simulink model "AB_Final_of_MPC_Bandwidth_Result_UnbalancedNew"  (R2022b)
settings: Solver=FixedStepDiscrete  StartTime=0.0  StopTime=Inf  FixedStep=100e-6  RelTol=1e-3  EnableMultiTasking=on
undefined symbols (not defined in the file): C28x, CPU1, CPU2, CurrentBypassValue, DiscIntNeverNeededParam, Down, GPTRIP1SEL, TZ1, Up
libraries: c2802xlib x20, simulink x17, dspstat3 x13, eeGeneralControl x10, c2837xDlib x5, c280xlib x5, PID_Lib x4, c2000lib x1, spsAlphaBetaZerotoabcLib x1
(part 4 of 10)

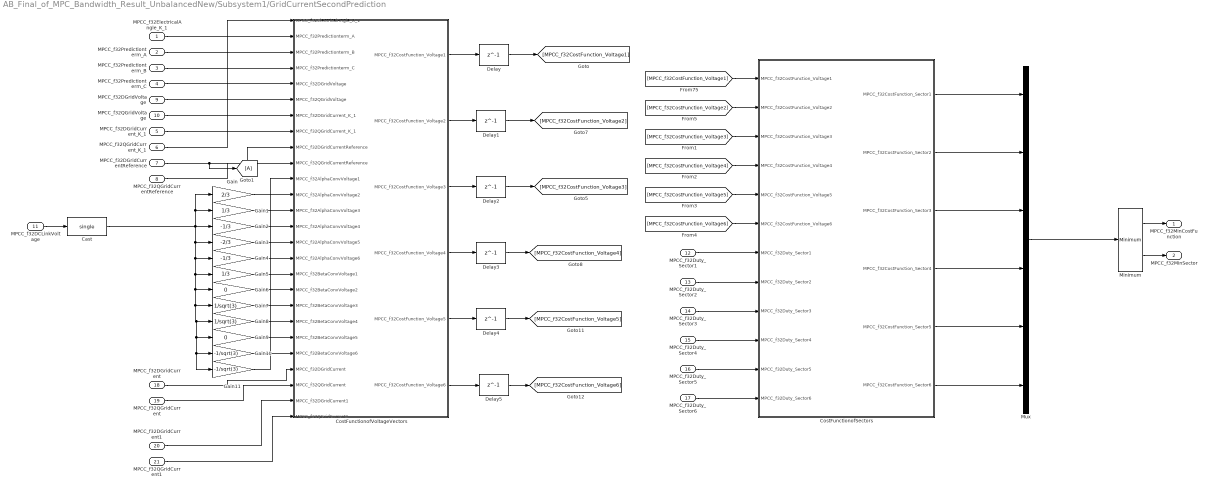
== system AB_Final_of_MPC_Bandwidth_Result_UnbalancedNew/Subsystem1/GridCurrentSecondPrediction ==
  MPCC_f32ElectricalAngle_K_1 : Inport
  MPCC_f32Predictionterm_A : Inport  Port=2
  MPCC_f32Predictionterm_B : Inport  Port=3
  MPCC_f32Predictionterm_C : Inport  Port=4
  MPCC_f32DGridCurrent_K_1 : Inport  Port=5
  MPCC_f32QGridCurrent_K_1 : Inport  Port=6
  MPCC_f32DGridCurrentReference : Inport  Port=7
  MPCC_f32QGridCurrentReference : Inport  Port=8
  MPCC_f32DGridVoltage : Inport  Port=9
  MPCC_f32QGridVoltage : Inport  Port=10
  MPCC_f32DCLinkVoltage : Inport  Port=11
  MPCC_f32Duty_Sector1 : Inport  Port=12
  MPCC_f32Duty_Sector2 : Inport  Port=13
  MPCC_f32Duty_Sector3 : Inport  Port=14
  MPCC_f32Duty_Sector4 : Inport  Port=15
  MPCC_f32Duty_Sector5 : Inport  Port=16
  MPCC_f32Duty_Sector6 : Inport  Port=17
  MPCC_f32DGridCurrent : Inport  Port=18
  MPCC_f32QGridCurrent : Inport  Port=19
  MPCC_f32DGridCurrent1 : Inport  Port=20
  MPCC_f32QGridCurrent1 : Inport  Port=21
  Cast : DataTypeConversion  OutDataTypeStr=single  SaturateOnIntegerOverflow=off  RndMeth=Floor
  CostFunctionofSectors : Subsystem
  CostFunctionofVoltageVectors : Subsystem
  Delay{,1..5} (6 alike) : Delay  DelayLength=1  InitialCondition=single(1000000)  UseCircularBuffer=on
  Gain : Gain  Gain=2/3
  Gain1 : Gain  Gain=1/3
  Gain10 : Gain  Gain=-1/sqrt(3)
  Gain11 : Gain  Gain=-1/sqrt(3)
  Gain2 : Gain  Gain=-1/3
  Gain3 : Gain  Gain=-2/3
  Gain4 : Gain  Gain=-1/3
  Gain5 : Gain  Gain=1/3
  Gain6 : Gain  Gain=0
  Gain7 : Gain  Gain=1/sqrt(3)
  Gain8 : Gain  Gain=1/sqrt(3)
  Gain9 : Gain  Gain=0
  Goto1 : Goto
  Minimum : dspstat3/Minimum  operation=minimum  fcn=Value and Index  indexBase=One  operateOver=Each column  Dimension=1  InputProcessing=Columns as channels (frame based)  reset=None  roiEnable=off  roiType=Rectangles  roiPortion=Entire ROI  roiOutput=Individual statistics for each ROI  roiFlag=off  roundingMode=Floor  overflowMode=off
  Mux : Mux  Inputs=6
  MPCC_f32MinCostFunction : Outport
  MPCC_f32MinSector : Outport  Port=2
  wires:
  CostFunctionofVoltageVectors/3(MPCC_f32CostFunction_Voltage3) -> Delay2/1
  CostFunctionofVoltageVectors/2(MPCC_f32CostFunction_Voltage2) -> Delay1/1
  CostFunctionofVoltageVectors/5(MPCC_f32CostFunction_Voltage5) -> Delay4/1
  CostFunctionofVoltageVectors/6(MPCC_f32CostFunction_Voltage6) -> Delay5/1
  CostFunctionofVoltageVectors/4(MPCC_f32CostFunction_Voltage4) -> Delay3/1
  CostFunctionofVoltageVectors/1(MPCC_f32CostFunction_Voltage1) -> Delay/1
  MPCC_f32ElectricalAngle_K_1/1 -> CostFunctionofVoltageVectors/1(MPCC_f32ElectricalAngle_K_1)
  MPCC_f32Predictionterm_A/1 -> CostFunctionofVoltageVectors/2(MPCC_f32Predictionterm_A)
  MPCC_f32Predictionterm_B/1 -> CostFunctionofVoltageVectors/3(MPCC_f32Predictionterm_B)
  MPCC_f32Predictionterm_C/1 -> CostFunctionofVoltageVectors/4(MPCC_f32Predictionterm_C)
  MPCC_f32DGridVoltage/1 -> CostFunctionofVoltageVectors/5(MPCC_f32DGridVoltage)
  MPCC_f32QGridVoltage/1 -> CostFunctionofVoltageVectors/6(MPCC_f32QGridVoltage)
  MPCC_f32DGridCurrent_K_1/1 -> CostFunctionofVoltageVectors/7(MPCC_f32DGridCurrent_K_1)
  MPCC_f32QGridCurrent_K_1/1 -> CostFunctionofVoltageVectors/8(MPCC_f32QGridCurrent_K_1)
  MPCC_f32DGridCurrentReference/1 -> Goto1/1, CostFunctionofVoltageVectors/9(MPCC_f32DGridCurrentReference)
  MPCC_f32QGridCurrentReference/1 -> CostFunctionofVoltageVectors/10(MPCC_f32QGridCurrentReference)
  MPCC_f32DCLinkVoltage/1 -> Cast/1
  Gain/1 -> CostFunctionofVoltageVectors/11(MPCC_f32AlphaConvVoltage1)
  Gain1/1 -> CostFunctionofVoltageVectors/12(MPCC_f32AlphaConvVoltage2)
  Gain2/1 -> CostFunctionofVoltageVectors/13(MPCC_f32AlphaConvVoltage3)
  Gain3/1 -> CostFunctionofVoltageVectors/14(MPCC_f32AlphaConvVoltage4)
  Gain4/1 -> CostFunctionofVoltageVectors/15(MPCC_f32AlphaConvVoltage5)
  Gain5/1 -> CostFunctionofVoltageVectors/16(MPCC_f32AlphaConvVoltage6)
  Gain6/1 -> CostFunctionofVoltageVectors/17(MPCC_f32BetaConvVoltage1)
  Gain7/1 -> CostFunctionofVoltageVectors/18(MPCC_f32BetaConvVoltage2)
  Gain8/1 -> CostFunctionofVoltageVectors/19(MPCC_f32BetaConvVoltage3)
  Gain9/1 -> CostFunctionofVoltageVectors/20(MPCC_f32BetaConvVoltage4)
  Gain10/1 -> CostFunctionofVoltageVectors/21(MPCC_f32BetaConvVoltage5)
  Gain11/1 -> CostFunctionofVoltageVectors/22(MPCC_f32BetaConvVoltage6)
  [MPCC_f32CostFunction_Voltage1] -> CostFunctionofSectors/1(MPCC_f32CostFunction_Voltage1)
  [MPCC_f32CostFunction_Voltage4] -> CostFunctionofSectors/4(MPCC_f32CostFunction_Voltage4)
  [MPCC_f32CostFunction_Voltage5] -> CostFunctionofSectors/5(MPCC_f32CostFunction_Voltage5)
  [MPCC_f32CostFunction_Voltage6] -> CostFunctionofSectors/6(MPCC_f32CostFunction_Voltage6)
  [MPCC_f32CostFunction_Voltage2] -> CostFunctionofSectors/2(MPCC_f32CostFunction_Voltage2)
  [MPCC_f32CostFunction_Voltage3] -> CostFunctionofSectors/3(MPCC_f32CostFunction_Voltage3)
  CostFunctionofSectors/1(MPCC_f32CostFunction_Sector1) -> Mux/1
  CostFunctionofSectors/2(MPCC_f32CostFunction_Sector2) -> Mux/2
  CostFunctionofSectors/3(MPCC_f32CostFunction_Sector3) -> Mux/3
  CostFunctionofSectors/4(MPCC_f32CostFunction_Sector4) -> Mux/4
  CostFunctionofSectors/5(MPCC_f32CostFunction_Sector5) -> Mux/5
  CostFunctionofSectors/6(MPCC_f32CostFunction_Sector6) -> Mux/6
  Mux/1 -> Minimum/1
  MPCC_f32Duty_Sector1/1 -> CostFunctionofSectors/7(MPCC_f32Duty_Sector1)
  MPCC_f32Duty_Sector2/1 -> CostFunctionofSectors/8(MPCC_f32Duty_Sector2)
  MPCC_f32Duty_Sector3/1 -> CostFunctionofSectors/9(MPCC_f32Duty_Sector3)
  MPCC_f32Duty_Sector4/1 -> CostFunctionofSectors/10(MPCC_f32Duty_Sector4)
  MPCC_f32Duty_Sector5/1 -> CostFunctionofSectors/11(MPCC_f32Duty_Sector5)
  MPCC_f32Duty_Sector6/1 -> CostFunctionofSectors/12(MPCC_f32Duty_Sector6)
  Cast/1 -> Gain4/1, Gain9/1, Gain11/1, Gain10/1, Gain8/1, Gain7/1, Gain6/1, Gain5/1, Gain3/1, Gain/1, Gain1/1, Gain2/1
  Delay/1 -> [MPCC_f32CostFunction_Voltage1]
  Delay1/1 -> [MPCC_f32CostFunction_Voltage2]
  Delay2/1 -> [MPCC_f32CostFunction_Voltage3]
  Delay3/1 -> [MPCC_f32CostFunction_Voltage4]
  Delay4/1 -> [MPCC_f32CostFunction_Voltage5]
  Delay5/1 -> [MPCC_f32CostFunction_Voltage6]
  MPCC_f32QGridCurrent/1 -> CostFunctionofVoltageVectors/24(MPCC_f32QGridCurrent)
  MPCC_f32DGridCurrent/1 -> CostFunctionofVoltageVectors/23(MPCC_f32DGridCurrent)
  Minimum/1 -> MPCC_f32MinCostFunction/1
  Minimum/2 -> MPCC_f32MinSector/1
  MPCC_f32DGridCurrent1/1 -> CostFunctionofVoltageVectors/25(MPCC_f32DGridCurrent1)
  MPCC_f32QGridCurrent1/1 -> CostFunctionofVoltageVectors/26(MPCC_f32QGridCurrent1)

== system AB_Final_of_MPC_Bandwidth_Result_UnbalancedNew/Subsystem1/ModulatorTimes ==
  MPCC_f32ElectricalAngle_K_1 : Inport
  MPCC_f32DCLinkVoltage : Inport  Port=2
  MPCC_f32Duty_Sector1 : Inport  Port=3
  MPCC_f32Duty_Sector2 : Inport  Port=4
  MPCC_f32Duty_Sector3 : Inport  Port=5
  MPCC_f32Duty_Sector4 : Inport  Port=6
  MPCC_f32Duty_Sector5 : Inport  Port=7
  MPCC_f32Duty_Sector6 : Inport  Port=8
  MPCC_f32MinSector : Inport  Port=9
  MPCC_f32SwitchingPeriod : Inport  Port=10
  Cast : DataTypeConversion  OutDataTypeStr=single  SaturateOnIntegerOverflow=off  RndMeth=Floor
  ConverterVoltage : Subsystem
  Gain : Gain  Gain=2/3
  Gain1 : Gain  Gain=1/3
  Gain10 : Gain  Gain=-1/sqrt(3)
  Gain11 : Gain  Gain=-1/sqrt(3)
  Gain2 : Gain  Gain=-1/3
  Gain3 : Gain  Gain=-2/3
  Gain4 : Gain  Gain=-1/3
  Gain5 : Gain  Gain=1/3
  Gain6 : Gain  Gain=0
  Gain7 : Gain  Gain=1/sqrt(3)
  Gain8 : Gain  Gain=1/sqrt(3)
  Gain9 : Gain  Gain=0
  ModulationVectorTimes : Subsystem
  MPCC_f32DQConvVoltage : Outport
  MPCC_f32Time1 : Outport  Port=2
  MPCC_f32Time2 : Outport  Port=3
  MPCC_f32Time0 : Outport  Port=4
  MPCC_u8ModulationSector : Outport  Port=5
  wires:
  MPCC_f32ElectricalAngle_K_1/1 -> ConverterVoltage/1(MPCC_f32ElectricalAngle_K_1)
  MPCC_f32DCLinkVoltage/1 -> Cast/1
  Gain/1 -> ConverterVoltage/2(MPCC_f32AlphaConvVoltage1)
  Gain1/1 -> ConverterVoltage/3(MPCC_f32AlphaConvVoltage2)
  Gain2/1 -> ConverterVoltage/4(MPCC_f32AlphaConvVoltage3)
  Gain3/1 -> ConverterVoltage/5(MPCC_f32AlphaConvVoltage4)
  Gain4/1 -> ConverterVoltage/6(MPCC_f32AlphaConvVoltage5)
  Gain5/1 -> ConverterVoltage/7(MPCC_f32AlphaConvVoltage6)
  Gain6/1 -> ConverterVoltage/8(MPCC_f32BetaConvVoltage1)
  Gain7/1 -> ConverterVoltage/9(MPCC_f32BetaConvVoltage2)
  Gain8/1 -> ConverterVoltage/10(MPCC_f32BetaConvVoltage3)
  Gain9/1 -> ConverterVoltage/11(MPCC_f32BetaConvVoltage4)
  Gain10/1 -> ConverterVoltage/12(MPCC_f32BetaConvVoltage5)
  Gain11/1 -> ConverterVoltage/13(MPCC_f32BetaConvVoltage6)
  ConverterVoltage/1(MPCC_f32DQConvVoltage) -> MPCC_f32DQConvVoltage/1
  MPCC_f32Duty_Sector5/1 -> [MPCC_f32Duty_Sector5]
  MPCC_f32Duty_Sector1/1 -> [MPCC_f32Duty_Sector1]
  MPCC_f32Duty_Sector6/1 -> [MPCC_f32Duty_Sector6]
  MPCC_f32Duty_Sector2/1 -> [MPCC_f32Duty_Sector2]
  MPCC_f32Duty_Sector4/1 -> [MPCC_f32Duty_Sector4]
  MPCC_f32Duty_Sector3/1 -> [MPCC_f32Duty_Sector3]
  MPCC_f32MinSector/1 -> [MPCC_f32MinSector], ConverterVoltage/20(MPCC_f32MinSector)
  [MPCC_f32Duty_Sector6] -> ConverterVoltage/19(MPCC_f32Duty_Sector6)
  [MPCC_f32Duty_Sector5] -> ConverterVoltage/18(MPCC_f32Duty_Sector5)
  [MPCC_f32Duty_Sector1] -> ConverterVoltage/14(MPCC_f32Duty_Sector1)
  [MPCC_f32Duty_Sector2] -> ConverterVoltage/15(MPCC_f32Duty_Sector2)
  [MPCC_f32Duty_Sector3] -> ConverterVoltage/16(MPCC_f32Duty_Sector3)
  [MPCC_f32Duty_Sector4] -> ConverterVoltage/17(MPCC_f32Duty_Sector4)
  [MPCC_f32Duty_Sector1] -> ModulationVectorTimes/1(MPCC_f32Duty_Sector1)
  [MPCC_f32Duty_Sector2] -> ModulationVectorTimes/2(MPCC_f32Duty_Sector2)
  [MPCC_f32Duty_Sector3] -> ModulationVectorTimes/3(MPCC_f32Duty_Sector3)
  [MPCC_f32Duty_Sector4] -> ModulationVectorTimes/4(MPCC_f32Duty_Sector4)
  [MPCC_f32Duty_Sector5] -> ModulationVectorTimes/5(MPCC_f32Duty_Sector5)
  [MPCC_f32Duty_Sector6] -> ModulationVectorTimes/6(MPCC_f32Duty_Sector6)
  MPCC_f32SwitchingPeriod/1 -> ModulationVectorTimes/7(MPCC_f32SwitchingPeriod)
  [MPCC_f32MinSector] -> ModulationVectorTimes/8(MPCC_f32MinSector)
  ModulationVectorTimes/3(MPCC_f32Time0) -> MPCC_f32Time0/1
  ModulationVectorTimes/1(MPCC_f32Time1) -> MPCC_f32Time1/1
  ModulationVectorTimes/2(MPCC_f32Time2) -> MPCC_f32Time2/1
  ModulationVectorTimes/4(MPCC_u8ModulationSector) -> MPCC_u8ModulationSector/1
  Cast/1 -> Gain/1, Gain4/1, Gain9/1, Gain11/1, Gain10/1, Gain8/1, Gain7/1, Gain6/1, Gain5/1, Gain3/1, Gain2/1, Gain1/1

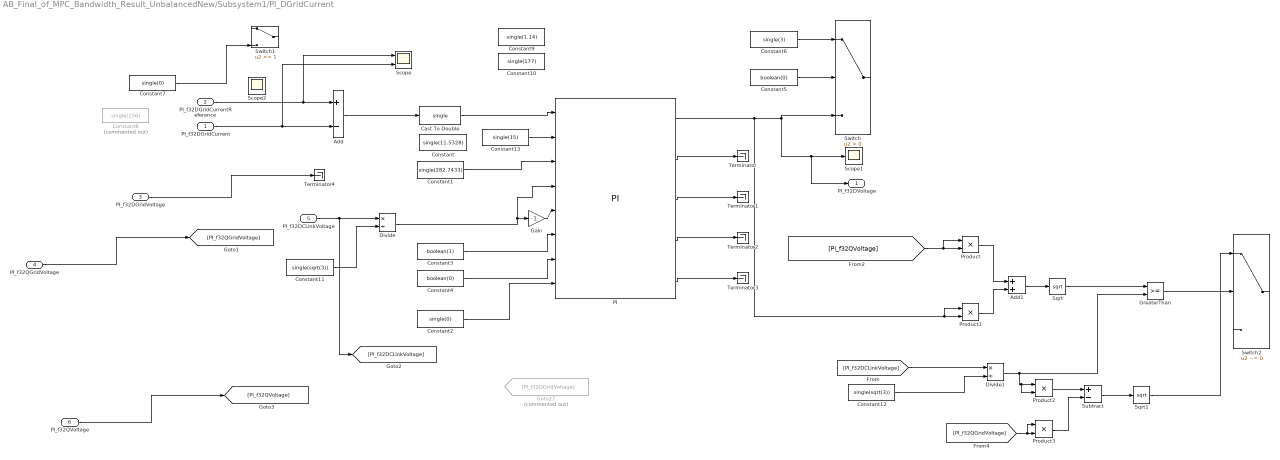
== system AB_Final_of_MPC_Bandwidth_Result_UnbalancedNew/Subsystem1/PI_DGridCurrent ==
  PI_f32DGridCurrent : Inport
  PI_f32DGridCurrentReference : Inport  Port=2
  PI_f32DGridVoltage : Inport  Port=3
  PI_f32QGridVoltage : Inport  Port=4
  PI_f32DCLinkVoltage : Inport  Port=5
  PI_f32QVoltage : Inport  Port=6
  Add : Sum  Inputs=+-
  Add1 : Sum
  Cast To Double : DataTypeConversion  OutDataTypeStr=single  SaturateOnIntegerOverflow=off  RndMeth=Floor
  Constant : Constant  Value=single(11.5328)
  Constant1 : Constant  Value=single(282.7433)
  Constant10 : Constant  Value=single(177)
  Constant11 : Constant  Value=single(sqrt(3))
  Constant12 : Constant  Value=single(sqrt(3))
  Constant13 : Constant  Value=single(15)
  Constant2 : Constant  Value=single(0)
  Constant3 : Constant  Value=boolean(1)
  Constant4 : Constant  Value=boolean(0)
  Constant5 : Constant  Value=boolean(0)
  Constant6 : Constant  Value=single(3)
  Constant7 : Constant  Value=single(0)
  Constant8 : Constant  Commented=on  Value=single(156)
  Constant9 : Constant  Value=single(1.14)
  Divide : Product  Inputs=*/  RndMeth=Zero  SaturateOnIntegerOverflow=on
  Divide1 : Product  Inputs=*/  RndMeth=Zero  SaturateOnIntegerOverflow=on
  Gain : Gain  Gain=-1
  Goto27 : Goto  Commented=on  GotoTag=PI_f32DGridVoltage
  GreaterThan : RelationalOperator  OutDataTypeStr=boolean  RndMeth=Simplest  InputSameDT=off
  PI : PID_Lib/PI  SystemSampleTime=-1  VariantActivationTime=update diagram  Latency=0  AutoFrameSizeCalculation=off
  Product{,1..3} (4 alike) : Product
  Scope : Scope  NumInputPorts=2
  Scope1 : Scope
  Scope2 : Scope
  Sqrt : Sqrt
  Sqrt1 : Sqrt
  Subtract : Sum  Inputs=+-
  Switch : Switch  Criteria=u2 > Threshold  SaturateOnIntegerOverflow=off  InputSameDT=off
  Switch1 : Switch  Threshold=1  SaturateOnIntegerOverflow=off  InputSameDT=off
  Switch2 : Switch  Criteria=u2 ~= 0  SaturateOnIntegerOverflow=off  InputSameDT=off
  Terminator{,1..4} (5 alike) : Terminator
  PI_f32DVoltage : Outport
  wires:
  PI_f32DGridCurrent/1 -> Scope/2, Add/2
  Gain/1 -> PI/5
  Constant3/1 -> PI/6
  Constant4/1 -> PI/7
  PI/2 -> Terminator/1
  PI/3 -> Terminator1/1
  PI/4 -> Terminator2/1
  PI/5 -> Terminator3/1
  Constant5/1 -> Switch/2
  Constant6/1 -> Switch/1
  Cast To Double/1 -> PI/1
  Add/1 -> Cast To Double/1
  Constant7/1 -> Switch1/3
  PI_f32DGridCurrentReference/1 -> Scope/1, Add/1
  Constant2/1 -> PI/8
  PI_f32DGridVoltage/1 -> Terminator4/1
  PI_f32QGridVoltage/1 -> [PI_f32QGridVoltage]
  Add1/1 -> Sqrt/1
  Product1/1 -> Add1/2
  Product/1 -> Add1/1
  [PI_f32QVoltage] -> Product/1, Product/2
  PI/1 -> Product1/1, Product1/2, Switch/3, PI_f32DVoltage/1, Scope1/1
  PI_f32DCLinkVoltage/1 -> [PI_f32DCLinkVoltage], Divide/1
  Constant11/1 -> Divide/2
  Constant12/1 -> Divide1/2
  [PI_f32DCLinkVoltage] -> Divide1/1
  Sqrt/1 -> GreaterThan/1
  Divide1/1 -> Product2/2, Product2/1, GreaterThan/2
  GreaterThan/1 -> Switch2/2
  Product2/1 -> Subtract/1
  [PI_f32QGridVoltage] -> Product3/1, Product3/2
  Product3/1 -> Subtract/2
  Subtract/1 -> Sqrt1/1
  Sqrt1/1 -> Switch2/1
  Divide/1 -> PI/4, Gain/1
  PI_f32QVoltage/1 -> [PI_f32QVoltage]
  Constant1/1 -> PI/3
  Constant13/1 -> PI/2

== system AB_Final_of_MPC_Bandwidth_Result_UnbalancedNew/Subsystem1/PI_QGridCurrent ==
  PI_f32QGridCurrentReference : Inport
  PI_f32QGridCurrent : Inport  Port=2
  PI_f32QGridVoltage : Inport  Port=3
  PI_f32DGridVoltage : Inport  Port=4
  PI_f32DCLinkVoltage : Inport  Port=5
  Add : Sum  Inputs=+-
  Add1 : Sum
  Cast To Single : DataTypeConversion  OutDataTypeStr=single  SaturateOnIntegerOverflow=off  RndMeth=Floor
  Constant : Constant  Value=single(11.5328)
  Constant1 : Constant  Value=single(282.7433)
  Constant10 : Constant  Value=single(177)
  Constant11 : Constant  Value=single(sqrt(3))
  Constant12 : Constant  Value=single(1.14)
  Constant13 : Constant  Value=single(sqrt(3))
  Constant14 : Constant  Value=single(15)
  Constant2 : Constant  Value=single(156)
  Constant3 : Constant  Value=boolean(1)
  Constant4 : Constant  Value=boolean(0)
  Constant5 : Constant  Value=boolean(0)
  Constant6 : Constant  Value=single(3)
  Constant7 : Constant  Value=single(0)
  Constant8 : Constant  Value=single(177)
  Constant9 : Constant  Value=single(1.14)
  Divide : Product  Inputs=*/  RndMeth=Zero  SaturateOnIntegerOverflow=on
  Divide1 : Product  Inputs=*/  RndMeth=Zero  SaturateOnIntegerOverflow=on
  Gain : Gain  Gain=-1
  PI : PID_Lib/PI  SystemSampleTime=-1  VariantActivationTime=update diagram  Latency=0  AutoFrameSizeCalculation=off
  Product{,1..3} (4 alike) : Product
  Sqrt : Sqrt
  Sqrt1 : Sqrt
  Subtract : Sum  Inputs=+-
  Switch : Switch  Criteria=u2 > Threshold  SaturateOnIntegerOverflow=off  InputSameDT=off
  Terminator{,1..4} (5 alike) : Terminator
  PI_f32QVoltage : Outport
  wires:
  PI_f32QGridCurrentReference/1 -> Add/1
  PI_f32QGridCurrent/1 -> Add/2
  Add/1 -> Cast To Single/1
  Gain/1 -> PI/5
  Constant3/1 -> PI/6
  Constant4/1 -> PI/7
  PI/2 -> Terminator/1
  PI/3 -> Terminator1/1
  PI/4 -> Terminator2/1
  PI/5 -> Terminator3/1
  Constant5/1 -> Switch/2
  Constant6/1 -> Switch/1
  Switch/1 -> PI_f32QVoltage/1
  Cast To Single/1 -> PI/1
  PI/1 -> Switch/3
  Constant7/1 -> PI/8
  PI_f32QGridVoltage/1 -> [PI_f32QGridVoltage]
  [PI_f32QGridVoltage] -> Terminator4/1
  PI_f32DGridVoltage/1 -> [PI_f32DGridVoltage]
  Product/1 -> Add1/1
  [PI_f32DGridVoltage] -> Product1/1, Product1/2
  [PI_f32QGridVoltage] -> Product/1, Product/2
  Product1/1 -> Add1/2
  Add1/1 -> Sqrt/1
  Constant11/1 -> Divide/2
  Subtract/1 -> Sqrt1/1
  [PI_f32DCLinkVoltage] -> Divide1/1
  [PI_f32DGridVoltage] -> Product3/1, Product3/2
  Product3/1 -> Subtract/2
  Product2/1 -> Subtract/1
  Divide1/1 -> Product2/2, Product2/1
  Constant13/1 -> Divide1/2
  PI_f32DCLinkVoltage/1 -> Divide/1, [PI_f32DCLinkVoltage]
  Divide/1 -> Gain/1, PI/4
  Constant1/1 -> PI/3
  Constant14/1 -> PI/2

== system AB_Final_of_MPC_Bandwidth_Result_UnbalancedNew/Subsystem1/PSCE ==
  w : Inport
  alpha : Inport  Port=2
  beta : Inport  Port=3
  Add5 : Sum  Inputs=+-
  Add6 : Sum
  Gain2 : Gain  Gain=0.5
  Gain3 : Gain  Gain=0.5
  SOGI 1st4 : Subsystem
  SOGI 1st5 : Subsystem
  alphap : Outport
  betap : Outport  Port=2
  Ealpha : Outport  Port=3
  betap1 : Outport  Port=4
  Ealpha_ : Outport  Port=5
  betap2 : Outport  Port=6
  Ebeta : Outport  Port=7
  Ebeta_ : Outport  Port=8
  wires:
  Add5/1 -> Gain2/1
  w/1 -> SOGI 1st5/1(w), SOGI 1st4/1(w)
  SOGI 1st5/1(v) -> betap1/1, Ebeta/1, Add6/1
  Gain3/1 -> betap/1
  SOGI 1st5/2(qv) -> Add5/2, Ebeta_/1, betap2/1
  alpha/1 -> SOGI 1st4/2(Vαβ)
  beta/1 -> SOGI 1st5/2(Vαβ)
  SOGI 1st4/1(v) -> Ealpha/1, Add5/1
  Add6/1 -> Gain3/1
  Gain2/1 -> alphap/1
  SOGI 1st4/2(qv) -> Ealpha_/1, Add6/2

== system AB_Final_of_MPC_Bandwidth_Result_UnbalancedNew/Subsystem1/PSCE1 ==
  w : Inport
  alpha : Inport  Port=2
  beta : Inport  Port=3
  Add5 : Sum  Inputs=+-
  Add6 : Sum
  Gain2 : Gain  Gain=0.5
  Gain3 : Gain  Gain=0.5
  SOGI 1st4 : Subsystem
  SOGI 1st5 : Subsystem
  alphap : Outport
  betap : Outport  Port=2
  alphan : Outport  Port=3
  betan : Outport  Port=4
  wires:
  Add5/1 -> Gain2/1
  w/1 -> SOGI 1st5/1(w), SOGI 1st4/1(w)
  SOGI 1st5/1(v) -> betap/1, Add6/1
  SOGI 1st5/2(qv) -> betan/1, Add5/2
  alpha/1 -> SOGI 1st4/2(Vαβ)
  beta/1 -> SOGI 1st5/2(Vαβ)
  SOGI 1st4/1(v) -> alphap/1, Add5/1
  Add6/1 -> Gain3/1
  SOGI 1st4/2(qv) -> alphan/1, Add6/2

== system AB_Final_of_MPC_Bandwidth_Result_UnbalancedNew/Subsystem1/SOGI 1st6 ==
  w : Inport
  Vαβ : Inport  Port=2
  Gain : Gain  Gain=sqrt(2)  OutDataTypeStr=single
  Gain1 : Gain  Gain=0  OutDataTypeStr=single
  Integrator : Subsystem
  Integrator1 : Subsystem
  Integrator2 : Subsystem
  Multiply : Product
  Multiply1 : Product
  Multiply2 : Product
  Saturation : Saturate  UpperLimit=5  LowerLimit=-5
  Sum : Sum  Inputs=-+|
  Sum1 : Sum  Inputs=|+-
  Sum2 : Sum  Inputs=++|
  v : Outport
  qv : Outport  Port=2  OutDataTypeStr=single
  wires:
  w/1 -> Multiply2/2, Multiply/2, Multiply1/1
  Sum/1 -> Saturation/1, Gain/1
  Gain/1 -> Sum1/1
  Vαβ/1 -> Sum/2
  Sum1/1 -> Multiply/1
  Multiply/1 -> Integrator/1(In)
  Multiply2/1 -> Integrator2/1(In)
  Gain1/1 -> Multiply2/1
  Saturation/1 -> Gain1/1
  Integrator/1(Out) -> Sum2/2, v/1, Integrator1/1(In)
  Integrator1/1(Out) -> Multiply1/2
  Multiply1/1 -> Sum1/2, qv/1
  Integrator2/1(Out) -> Sum2/1
  Sum2/1 -> Sum/1

== system AB_Final_of_MPC_Bandwidth_Result_UnbalancedNew/Subsystem1/SOGI 1st7 ==
  w : Inport
  Vαβ : Inport  Port=2
  Gain : Gain  Gain=sqrt(2)  OutDataTypeStr=single
  Gain1 : Gain  Gain=0  OutDataTypeStr=single
  Integrator : Subsystem
  Integrator1 : Subsystem
  Integrator2 : Subsystem
  Multiply : Product
  Multiply1 : Product
  Multiply2 : Product
  Saturation : Saturate  UpperLimit=5  LowerLimit=-5
  Sum : Sum  Inputs=-+|
  Sum1 : Sum  Inputs=|+-
  Sum2 : Sum  Inputs=++|
  v : Outport
  qv : Outport  Port=2  OutDataTypeStr=single
  wires:
  w/1 -> Multiply2/2, Multiply/2, Multiply1/1
  Sum/1 -> Saturation/1, Gain/1
  Gain/1 -> Sum1/1
  Vαβ/1 -> Sum/2
  Sum1/1 -> Multiply/1
  Multiply/1 -> Integrator/1(In)
  Multiply2/1 -> Integrator2/1(In)
  Gain1/1 -> Multiply2/1
  Saturation/1 -> Gain1/1
  Integrator/1(Out) -> Sum2/2, v/1, Integrator1/1(In)
  Integrator1/1(Out) -> Multiply1/2
  Multiply1/1 -> Sum1/2, qv/1
  Integrator2/1(Out) -> Sum2/1
  Sum2/1 -> Sum/1

== system AB_Final_of_MPC_Bandwidth_Result_UnbalancedNew/Subsystem1/SOGI 1st8 ==
  w : Inport
  Vαβ : Inport  Port=2
  Gain : Gain  Gain=sqrt(2)  OutDataTypeStr=single
  Gain1 : Gain  Gain=0  OutDataTypeStr=single
  Integrator : Subsystem
  Integrator1 : Subsystem
  Integrator2 : Subsystem
  Multiply : Product
  Multiply1 : Product
  Multiply2 : Product
  Saturation : Saturate  UpperLimit=5  LowerLimit=-5
  Sum : Sum  Inputs=-+|
  Sum1 : Sum  Inputs=|+-
  Sum2 : Sum  Inputs=++|
  v : Outport
  qv : Outport  Port=2  OutDataTypeStr=single
  wires:
  w/1 -> Multiply2/2, Multiply/2, Multiply1/1
  Sum/1 -> Saturation/1, Gain/1
  Gain/1 -> Sum1/1
  Vαβ/1 -> Sum/2
  Sum1/1 -> Multiply/1
  Multiply/1 -> Integrator/1(In)
  Multiply2/1 -> Integrator2/1(In)
  Gain1/1 -> Multiply2/1
  Saturation/1 -> Gain1/1
  Integrator/1(Out) -> Sum2/2, v/1, Integrator1/1(In)
  Integrator1/1(Out) -> Multiply1/2
  Multiply1/1 -> Sum1/2, qv/1
  Integrator2/1(Out) -> Sum2/1
  Sum2/1 -> Sum/1

== system AB_Final_of_MPC_Bandwidth_Result_UnbalancedNew/Subsystem1/SOGI 1st9 ==
  w : Inport
  Vαβ : Inport  Port=2
  Gain : Gain  Gain=sqrt(2)  OutDataTypeStr=single
  Gain1 : Gain  Gain=0  OutDataTypeStr=single
  Integrator : Subsystem
  Integrator1 : Subsystem
  Integrator2 : Subsystem
  Multiply : Product
  Multiply1 : Product
  Multiply2 : Product
  Saturation : Saturate  UpperLimit=5  LowerLimit=-5
  Sum : Sum  Inputs=-+|
  Sum1 : Sum  Inputs=|+-
  Sum2 : Sum  Inputs=++|
  v : Outport
  qv : Outport  Port=2  OutDataTypeStr=single
  wires:
  w/1 -> Multiply2/2, Multiply/2, Multiply1/1
  Sum/1 -> Saturation/1, Gain/1
  Gain/1 -> Sum1/1
  Vαβ/1 -> Sum/2
  Sum1/1 -> Multiply/1
  Multiply/1 -> Integrator/1(In)
  Multiply2/1 -> Integrator2/1(In)
  Gain1/1 -> Multiply2/1
  Saturation/1 -> Gain1/1
  Integrator/1(Out) -> Sum2/2, v/1, Integrator1/1(In)
  Integrator1/1(Out) -> Multiply1/2
  Multiply1/1 -> Sum1/2, qv/1
  Integrator2/1(Out) -> Sum2/1
  Sum2/1 -> Sum/1

== system AB_Final_of_MPC_Bandwidth_Result_UnbalancedNew/Subsystem1/SVM ==
  Vabc : Inport
  Vdc : Inport  Port=2
  Add : Sum
  Add1 : Sum
  Constant1 : Constant
  Divide : Product  Inputs=*/
  Gain : Gain  Gain=uint32(5000)
  Gain2 : Gain  Gain=0.5
  Gain8 : Gain  Gain=0.5
  Gain9 : Gain  Gain=0.5
  Max : MinMax  Function=max
  Max1 : MinMax
  Saturation : Saturate  UpperLimit=single(2/sqrt(3))  LowerLimit=single(-2/sqrt(3))
  Saturation1 : Saturate  UpperLimit=5000  LowerLimit=0
  Subtract : Sum  Inputs=+-
  Dabc : Outport
  wires:
  Max/1 -> Add/1
  Gain8/1 -> Divide/2
  Add1/1 -> Gain9/1
  Add/1 -> Gain2/1
  Vabc/1 -> Subtract/1, Max1/1, Max/1
  Max1/1 -> Add/2
  Divide/1 -> Saturation/1
  Constant1/1 -> Add1/2
  Gain2/1 -> Subtract/2
  Subtract/1 -> Divide/1
  Gain9/1 -> Gain/1
  Vdc/1 -> Gain8/1
  Saturation/1 -> Add1/1
  Gain/1 -> Saturation1/1
  Saturation1/1 -> Dabc/1

== system AB_Final_of_MPC_Bandwidth_Result_UnbalancedNew/Subsystem1/SVPWM ==
  Valpha_beta : Inport
  Constant : Constant  Value=0.5  OutDataTypeStr=single
  Constant1 : Constant  Value=0.5  OutDataTypeStr=single
  Constant2 : Constant  Value=0.5  OutDataTypeStr=single
  Demux : Demux  Outputs=2
  Gain : Gain  Gain=uint32(5000)
  Gain{1,3..5} (4 alike) : Gain  Gain=0.5
  Gain2 : Gain  Gain=1/sqrt(3)
  Gain6 : Gain  Gain=uint32(5000)
  Gain7 : Gain  Gain=uint32(5000)
  Max : MinMax  Function=max  Inputs=3
  Min : MinMax  Inputs=3
  Sum{,1,7..9} (5 alike) : Sum  Inputs=|++
  Sum2 : Sum  Inputs=|-+
  Sum3 : Sum  Inputs=|--
  Sum4 : Sum  Inputs=|+-
  Sum5 : Sum  Inputs=|+-
  Sum6 : Sum  Inputs=|+-
  Da : Outport  VectorParamsAs1DForOutWhenUnconnected=off
  Db : Outport  Port=2  VectorParamsAs1DForOutWhenUnconnected=off
  Dc : Outport  Port=3  VectorParamsAs1DForOutWhenUnconnected=off
  wires:
  Gain5/1 -> Sum9/1
  Gain4/1 -> Sum8/1
  Gain1/1 -> Sum/1
  Valpha_beta/1 -> Demux/1
  Demux/2 -> Sum2/2, Sum3/2
  Demux/1 -> Gain2/1
  Sum9/1 -> Gain7/1
  Sum8/1 -> Gain6/1
  Sum/1 -> Gain/1
  Constant2/1 -> Sum9/2
  Constant1/1 -> Sum8/2
  Constant/1 -> Sum/2
  Gain3/1 -> Sum4/2, Sum5/2, Sum6/2
  Sum3/1 -> Max/3, Min/3, Sum6/1
  Sum1/1 -> Max/1, Min/1, Sum4/1
  Max/1 -> Sum7/1
  Sum7/1 -> Gain3/1
  Min/1 -> Sum7/2
  Sum2/1 -> Max/2, Sum5/1, Min/2
  Gain2/1 -> Sum1/1, Sum1/2, Sum2/1, Sum3/1
  Sum4/1 -> Gain1/1
  Sum5/1 -> Gain4/1
  Sum6/1 -> Gain5/1
  Gain/1 -> Da/1
  Gain6/1 -> Db/1
  Gain7/1 -> Dc/1

== system AB_Final_of_MPC_Bandwidth_Result_UnbalancedNew/Subsystem1/Start1 ==
  Data : Inport
  Data_width : Inport  Port=2
  Action Port : ActionPort  ActionPortLabel=if(u1 == 0)
  Bias : Bias  Bias=1  SaturateOnIntegerOverflow=off
  End : Constant  Value=hex2dec('5353')  OutDataTypeStr=uint16
  Mux : Mux  Inputs=2
  Data_out : Outport  VectorParamsAs1DForOutWhenUnconnected=off
  Iteration : Outport  Port=2  VectorParamsAs1DForOutWhenUnconnected=off
  wires:
  End/1 -> Mux/1
  Mux/1 -> Data_out/1
  Data_width/1 -> Bias/1
  Bias/1 -> Iteration/1
  Data/1 -> Mux/2

== system AB_Final_of_MPC_Bandwidth_Result_UnbalancedNew/Subsystem1/Subsystem ==
  PWM1 : Inport
  PWM2 : Inport  Port=2
  PWM3 : Inport  Port=3
  Trip : Inport  Port=4
  Constant12 : Constant  Value=uint32(4999)
  Constant13 : Constant  Value=uint32(0)
  Constant16 : Constant  Value=uint32(4999)
  Constant17 : Constant  Value=uint32(0)
  Constant6 : Constant  Value=uint32(4999)
  Constant7 : Constant  Value=uint32(0)
  Data Type Conversion18 : DataTypeConversion  OutDataTypeStr=uint32  SaturateOnIntegerOverflow=off  RndMeth=Floor
  Data Type Conversion19 : DataTypeConversion  OutDataTypeStr=uint32  SaturateOnIntegerOverflow=off  RndMeth=Floor
  Data Type Conversion5 : DataTypeConversion  OutDataTypeStr=uint32  SaturateOnIntegerOverflow=off  RndMeth=Floor
  From : From
  From1 : From
  From2 : From
  Gain : Gain
  Goto : Goto
  Saturation Dynamic1 : simulink/Discontinuities/Saturation Dynamic  OutMin=[]  OutMax=[]  OutDataTypeStr=Inherit: Same as second input  OutDataType=fixdt(1, 16)  OutScaling=2^-10  DoSatur=off
  Saturation Dynamic2 : simulink/Discontinuities/Saturation Dynamic  OutMin=[]  OutMax=[]  OutDataTypeStr=Inherit: Same as second input  OutDataType=fixdt(1, 16)  OutScaling=2^-10  DoSatur=off
  Saturation Dynamic3 : simulink/Discontinuities/Saturation Dynamic  OutMin=[]  OutMax=[]  OutDataTypeStr=Inherit: Same as second input  OutDataType=fixdt(1, 16)  OutScaling=2^-10  DoSatur=off
  ePWM5 : c2802xlib/ePWM  PwmType=C2000_Type4  useModule=ePWM1  ePWMxLINKTBPRD=Not Linked  periodUnits=Clock cycles  timerSource=Specify via dialog  timerPeriod_clk=5000  timerPeriod_sec=0.0001  tbshadow=Counter equals to zero  countingMode=Up-Down  phaseActiveEnable=Disable  phaseDirection=Count down after sync  phaseActive=0  synchronizationEnable=off  dcaevt1Sync=off  dcbevt1Sync=off  synchronizationOption=Disable  dcbevt1SyncOut=off  dcaevt1SyncOut=off  cmpdSyncOut=off  cmpcSyncOut=off  cmpbSyncOut=off  zeroSyncOut=off  swfSyncOut=off  perSynchronizationOption=Counter equals to period (CTR=PRD)  clockPrescale=1  HSclockPrescale=1  enswap=off  ePWMxAStatus=on  ePWMxAactionLogic1=Do nothing  ePWMxAactionLogic2=Do nothing  ePWMxAactionLogic3=Clear  ePWMxAactionLogic4=Set  ePWMxAactionLogic5=Do nothing  ePWMxAactionLogic6=Do nothing  ePWMxACSFenable=off  ePWMxACSFvalue=Forcing disable  ePWMxASFreload=Zero  ePWMxBStatus=off  ePWMxBactionLogic1=Set  ePWMxBactionLogic2=Clear  ePWMxBactionLogic3=Do nothing  ePWMxBactionLogic4=Do nothing  ePWMxBactionLogic5=Clear  ePWMxBactionLogic6=Set  ePWMxBCSFenable=off  ePWMxBCSFvalue=Forcing disable  ePWMxBSFreload=Zero  ePWNxBOutWay=off  ePWMxLINKCMPA=Not Linked  CMPAUnits=Clock cycles  CMPASource=Input port  CMPAValue_per=50  CMPAValue_clk=0  enCMPAshadow=Counter equals to zero (CTR=Zero)  ePWMxLINKCMPB=Not Linked  CMPBUnits=Clock cycles  CMPBSource=Specify via dialog  CMPBValue_per=50  CMPBValue_clk=0  enCMPBshadow=Counter equals to zero (CTR=Zero)  ePWMxLINKCMPC=Not Linked  CMPCUnits=Clock cycles  CMPCSource=Specify via dialog  CMPCValue_per=50  CMPCValue_clk=0  enCMPCshadow=Counter equals to zero (CTR=Zero)  ePWMxLINKCMPD=Not Linked  CMPDUnits=Clock cycles  CMPDSource=Specify via dialog  CMPDValue_per=50  CMPDValue_clk=0  enCMPDshadow=Counter equals to zero (CTR=Zero)  enableDBePWMxA=on  enableDBePWMxB=on  enhalfcycle=off  DBpolarity=Active high complementary (AHC)  DBedgeDelay=Positive  DBSource_ePWMxA=ePWMxA  DBSource_ePWMxB=ePWMxA  DBPeriodUnits=Seconds  DBperiodSource=Specify via dialog  REDperiod=250  FEDperiod=250  REDperiod_sec=500e-9  FEDperiod_sec=500e-9  LoadModeDBRED=Immediate without using shadow  LoadModeDBFED=Immediate without using shadow  adcstartModuleA=on  adcrequestEventA=First event  adcstartEventA=Digital Compare Module A Event 1 start of conversion (DCAEVT1.soc)  adcstartEventA_type2=Counter equals to period (CTR=PRD)  adcstartModuleB=off  adcrequestEventB=First event  adcstartEventB=Counter equals to zero (CTR=Zero)  adcstartEventB_type2=Counter equals to zero (CTR=Zero)  intEn=off  intPrd=First event  intSel=Counter equals to zero (CTR=Zero)  intSel_type2=Counter equals to zero (CTR=Zero)  hrpe=off  enHRPWM=off  HRPWM_LoadMode=Counter equals to period (CTR=PRD)  HRPWM_CTLMode=Duty or Period control mode  HRPWM_EDGMode=Both edge  hrpeb=off  enHRPWMB=off  HRPWM_LoadModeB=Counter equals to zero (CTR=ZERO)  HRPWM_CTLModeB=Duty or Period control mode  HRPWM_EDGModeB=Both edge  enHRDBRED=off  enHRDBFED=off  enSFO=on  enautoconv=on  chopperEnable=off  chopperFrequency=1  chopperFirstwidth=1  chopperDuty=12.5%  tripZonesource=Input port  tzselOSHT1=off  tzselOSHT2=off  tzselOSHT3=off  tzselOSHDCAEV1=off  tzselOSHDCBEV1=off  tzselCBC1=off  tzselCBC2=off  tzselCBC3=off  tzselCBCDCAEV2=off  tzselCBCDCBEV2=off  tzselOSHT4=off  tzselOSHT5=off  tzselOSHT6=off  tzselCBC4=off  tzselCBC5=off  tzselCBC6=off  enTzOstIntr=off  enTzCbcIntr=off  enTzDCAEVT1Intr=off  enTzDCAEVT2Intr=off  enTzDCBEVT1Intr=off  enTzDCBEVT2Intr=off  ePWMxAforced=Low  ePWMxBforced=Low  DCAEVT1forced=No action  DCBEVT1forced=No action  DCAEVT2forced=No action  DCBEVT2forced=No action  dcah=Trip Zone 1 input (TZ1)  dcal=Trip Zone 2 input (TZ2)  dcbh=Trip Zone 1 input (TZ1)  dcbl=Trip Zone 2 input (TZ2)  dcah_type2=GPTRIP1SEL/(TZ1)  dcal_type2=GPTRIP1SEL/(TZ1)  dcbh_type2=GPTRIP1SEL/(TZ1)  dcbl_type2=GPTRIP1SEL/(TZ1)  gendcaevt1=Event disabled  gendcaevt2=Event disabled  gendcbevt1=Event disabled  gendcbevt2=Event disabled  dcaevt1src=DCAEVT1 with sync  dcaevt2src=DCAEVT2 with sync  dcbevt1src=DCBEVT1 with sync  dcbevt2src=DCBEVT2 with sync  pulsesel=Counter equals to zero (CTR=Zero)  blankinv=off  blankoffset=0  blankwidth=0  evsrcsel=Filtered version of DCAEVT1 (DCAEVT1FILT)  encape=off
  ePWM6 : c2802xlib/ePWM  PwmType=C2000_Type4  useModule=ePWM2  ePWMxLINKTBPRD=Not Linked  periodUnits=Clock cycles  timerSource=Specify via dialog  timerPeriod_clk=5000  timerPeriod_sec=0.0001  tbshadow=Counter equals to zero  countingMode=Up-Down  phaseActiveEnable=Disable  phaseDirection=Count down after sync  phaseActive=0  synchronizationEnable=off  dcaevt1Sync=off  dcbevt1Sync=off  synchronizationOption=Disable  dcbevt1SyncOut=off  dcaevt1SyncOut=off  cmpdSyncOut=off  cmpcSyncOut=off  cmpbSyncOut=off  zeroSyncOut=off  swfSyncOut=off  perSynchronizationOption=Counter equals to period (CTR=PRD)  clockPrescale=1  HSclockPrescale=1  enswap=off  ePWMxAStatus=on  ePWMxAactionLogic1=Do nothing  ePWMxAactionLogic2=Do nothing  ePWMxAactionLogic3=Clear  ePWMxAactionLogic4=Set  ePWMxAactionLogic5=Do nothing  ePWMxAactionLogic6=Do nothing  ePWMxACSFenable=off  ePWMxACSFvalue=Forcing disable  ePWMxASFreload=Zero  ePWMxBStatus=off  ePWMxBactionLogic1=Set  ePWMxBactionLogic2=Clear  ePWMxBactionLogic3=Do nothing  ePWMxBactionLogic4=Do nothing  ePWMxBactionLogic5=Clear  ePWMxBactionLogic6=Set  ePWMxBCSFenable=off  ePWMxBCSFvalue=Forcing disable  ePWMxBSFreload=Zero  ePWNxBOutWay=off  ePWMxLINKCMPA=Not Linked  CMPAUnits=Clock cycles  CMPASource=Input port  CMPAValue_per=50  CMPAValue_clk=0  enCMPAshadow=Counter equals to zero (CTR=Zero)  ePWMxLINKCMPB=Not Linked  CMPBUnits=Clock cycles  CMPBSource=Specify via dialog  CMPBValue_per=50  CMPBValue_clk=0  enCMPBshadow=Counter equals to zero (CTR=Zero)  ePWMxLINKCMPC=Not Linked  CMPCUnits=Clock cycles  CMPCSource=Specify via dialog  CMPCValue_per=50  CMPCValue_clk=0  enCMPCshadow=Counter equals to zero (CTR=Zero)  ePWMxLINKCMPD=Not Linked  CMPDUnits=Clock cycles  CMPDSource=Specify via dialog  CMPDValue_per=50  CMPDValue_clk=0  enCMPDshadow=Counter equals to zero (CTR=Zero)  enableDBePWMxA=on  enableDBePWMxB=on  enhalfcycle=off  DBpolarity=Active high complementary (AHC)  DBedgeDelay=Positive  DBSource_ePWMxA=ePWMxA  DBSource_ePWMxB=ePWMxA  DBPeriodUnits=Seconds  DBperiodSource=Specify via dialog  REDperiod=250  FEDperiod=250  REDperiod_sec=500e-9  FEDperiod_sec=500e-9  LoadModeDBRED=Immediate without using shadow  LoadModeDBFED=Immediate without using shadow  adcstartModuleA=off  adcrequestEventA=First event  adcstartEventA=Digital Compare Module A Event 1 start of conversion (DCAEVT1.soc)  adcstartEventA_type2=Counter equals to zero (CTR=Zero)  adcstartModuleB=off  adcrequestEventB=First event  adcstartEventB=Counter equals to zero (CTR=Zero)  adcstartEventB_type2=Counter equals to zero (CTR=Zero)  intEn=off  intPrd=First event  intSel=Counter equals to zero (CTR=Zero)  intSel_type2=Counter equals to zero (CTR=Zero)  hrpe=off  enHRPWM=off  HRPWM_LoadMode=Counter equals to period (CTR=PRD)  HRPWM_CTLMode=Duty or Period control mode  HRPWM_EDGMode=Both edge  hrpeb=off  enHRPWMB=off  HRPWM_LoadModeB=Counter equals to zero (CTR=ZERO)  HRPWM_CTLModeB=Duty or Period control mode  HRPWM_EDGModeB=Both edge  enHRDBRED=off  enHRDBFED=off  enSFO=on  enautoconv=on  chopperEnable=off  chopperFrequency=1  chopperFirstwidth=1  chopperDuty=12.5%  tripZonesource=Input port  tzselOSHT1=off  tzselOSHT2=off  tzselOSHT3=off  tzselOSHDCAEV1=off  tzselOSHDCBEV1=off  tzselCBC1=off  tzselCBC2=off  tzselCBC3=off  tzselCBCDCAEV2=off  tzselCBCDCBEV2=off  tzselOSHT4=off  tzselOSHT5=off  tzselOSHT6=off  tzselCBC4=off  tzselCBC5=off  tzselCBC6=off  enTzOstIntr=off  enTzCbcIntr=off  enTzDCAEVT1Intr=off  enTzDCAEVT2Intr=off  enTzDCBEVT1Intr=off  enTzDCBEVT2Intr=off  ePWMxAforced=Low  ePWMxBforced=Low  DCAEVT1forced=No action  DCBEVT1forced=No action  DCAEVT2forced=No action  DCBEVT2forced=No action  dcah=Trip Zone 1 input (TZ1)  dcal=Trip Zone 2 input (TZ2)  dcbh=Trip Zone 1 input (TZ1)  dcbl=Trip Zone 2 input (TZ2)  dcah_type2=GPTRIP1SEL/(TZ1)  dcal_type2=GPTRIP1SEL/(TZ1)  dcbh_type2=GPTRIP1SEL/(TZ1)  dcbl_type2=GPTRIP1SEL/(TZ1)  gendcaevt1=Event disabled  gendcaevt2=Event disabled  gendcbevt1=Event disabled  gendcbevt2=Event disabled  dcaevt1src=DCAEVT1 with sync  dcaevt2src=DCAEVT2 with sync  dcbevt1src=DCBEVT1 with sync  dcbevt2src=DCBEVT2 with sync  pulsesel=Counter equals to zero (CTR=Zero)  blankinv=off  blankoffset=0  blankwidth=0  evsrcsel=Filtered version of DCAEVT1 (DCAEVT1FILT)  encape=off
  ePWM7 : c2802xlib/ePWM  PwmType=C2000_Type4  useModule=ePWM3  ePWMxLINKTBPRD=Not Linked  periodUnits=Clock cycles  timerSource=Specify via dialog  timerPeriod_clk=5000  timerPeriod_sec=0.0001  tbshadow=Counter equals to zero  countingMode=Up-Down  phaseActiveEnable=Disable  phaseDirection=Count down after sync  phaseActive=0  synchronizationEnable=off  dcaevt1Sync=off  dcbevt1Sync=off  synchronizationOption=Disable  dcbevt1SyncOut=off  dcaevt1SyncOut=off  cmpdSyncOut=off  cmpcSyncOut=off  cmpbSyncOut=off  zeroSyncOut=off  swfSyncOut=off  perSynchronizationOption=Counter equals to period (CTR=PRD)  clockPrescale=1  HSclockPrescale=1  enswap=off  ePWMxAStatus=on  ePWMxAactionLogic1=Do nothing  ePWMxAactionLogic2=Do nothing  ePWMxAactionLogic3=Clear  ePWMxAactionLogic4=Set  ePWMxAactionLogic5=Do nothing  ePWMxAactionLogic6=Do nothing  ePWMxACSFenable=off  ePWMxACSFvalue=Forcing disable  ePWMxASFreload=Zero  ePWMxBStatus=off  ePWMxBactionLogic1=Set  ePWMxBactionLogic2=Clear  ePWMxBactionLogic3=Do nothing  ePWMxBactionLogic4=Do nothing  ePWMxBactionLogic5=Clear  ePWMxBactionLogic6=Set  ePWMxBCSFenable=off  ePWMxBCSFvalue=Forcing disable  ePWMxBSFreload=Zero  ePWNxBOutWay=off  ePWMxLINKCMPA=Not Linked  CMPAUnits=Clock cycles  CMPASource=Input port  CMPAValue_per=50  CMPAValue_clk=0  enCMPAshadow=Counter equals to zero (CTR=Zero)  ePWMxLINKCMPB=Not Linked  CMPBUnits=Clock cycles  CMPBSource=Specify via dialog  CMPBValue_per=50  CMPBValue_clk=0  enCMPBshadow=Counter equals to zero (CTR=Zero)  ePWMxLINKCMPC=Not Linked  CMPCUnits=Clock cycles  CMPCSource=Specify via dialog  CMPCValue_per=50  CMPCValue_clk=0  enCMPCshadow=Counter equals to zero (CTR=Zero)  ePWMxLINKCMPD=Not Linked  CMPDUnits=Clock cycles  CMPDSource=Specify via dialog  CMPDValue_per=50  CMPDValue_clk=0  enCMPDshadow=Counter equals to zero (CTR=Zero)  enableDBePWMxA=on  enableDBePWMxB=on  enhalfcycle=off  DBpolarity=Active high complementary (AHC)  DBedgeDelay=Positive  DBSource_ePWMxA=ePWMxA  DBSource_ePWMxB=ePWMxA  DBPeriodUnits=Seconds  DBperiodSource=Specify via dialog  REDperiod=250  FEDperiod=250  REDperiod_sec=500e-9  FEDperiod_sec=500e-9  LoadModeDBRED=Immediate without using shadow  LoadModeDBFED=Immediate without using shadow  adcstartModuleA=off  adcrequestEventA=First event  adcstartEventA=Digital Compare Module A Event 1 start of conversion (DCAEVT1.soc)  adcstartEventA_type2=Counter equals to zero (CTR=Zero)  adcstartModuleB=off  adcrequestEventB=First event  adcstartEventB=Counter equals to zero (CTR=Zero)  adcstartEventB_type2=Counter equals to zero (CTR=Zero)  intEn=off  intPrd=First event  intSel=Counter equals to zero (CTR=Zero)  intSel_type2=Counter equals to zero (CTR=Zero)  hrpe=off  enHRPWM=off  HRPWM_LoadMode=Counter equals to period (CTR=PRD)  HRPWM_CTLMode=Duty or Period control mode  HRPWM_EDGMode=Both edge  hrpeb=off  enHRPWMB=off  HRPWM_LoadModeB=Counter equals to zero (CTR=ZERO)  HRPWM_CTLModeB=Duty or Period control mode  HRPWM_EDGModeB=Both edge  enHRDBRED=off  enHRDBFED=off  enSFO=on  enautoconv=on  chopperEnable=off  chopperFrequency=1  chopperFirstwidth=1  chopperDuty=12.5%  tripZonesource=Input port  tzselOSHT1=off  tzselOSHT2=off  tzselOSHT3=off  tzselOSHDCAEV1=off  tzselOSHDCBEV1=off  tzselCBC1=off  tzselCBC2=off  tzselCBC3=off  tzselCBCDCAEV2=off  tzselCBCDCBEV2=off  tzselOSHT4=off  tzselOSHT5=off  tzselOSHT6=off  tzselCBC4=off  tzselCBC5=off  tzselCBC6=off  enTzOstIntr=off  enTzCbcIntr=off  enTzDCAEVT1Intr=off  enTzDCAEVT2Intr=off  enTzDCBEVT1Intr=off  enTzDCBEVT2Intr=off  ePWMxAforced=Low  ePWMxBforced=Low  DCAEVT1forced=No action  DCBEVT1forced=No action  DCAEVT2forced=No action  DCBEVT2forced=No action  dcah=Trip Zone 1 input (TZ1)  dcal=Trip Zone 2 input (TZ2)  dcbh=Trip Zone 1 input (TZ1)  dcbl=Trip Zone 2 input (TZ2)  dcah_type2=GPTRIP1SEL/(TZ1)  dcal_type2=GPTRIP1SEL/(TZ1)  dcbh_type2=GPTRIP1SEL/(TZ1)  dcbl_type2=GPTRIP1SEL/(TZ1)  gendcaevt1=Event disabled  gendcaevt2=Event disabled  gendcbevt1=Event disabled  gendcbevt2=Event disabled  dcaevt1src=DCAEVT1 with sync  dcaevt2src=DCAEVT2 with sync  dcbevt1src=DCBEVT1 with sync  dcbevt2src=DCBEVT2 with sync  pulsesel=Counter equals to zero (CTR=Zero)  blankinv=off  blankoffset=0  blankwidth=0  evsrcsel=Filtered version of DCAEVT1 (DCAEVT1FILT)  encape=off
  wires:
  Data Type Conversion5/1 -> ePWM5/1
  Constant13/1 -> Saturation Dynamic3/3
  Constant6/1 -> Saturation Dynamic1/1
  Constant12/1 -> Saturation Dynamic3/1
  Constant7/1 -> Saturation Dynamic1/3
  Saturation Dynamic1/1 -> Data Type Conversion5/1
  Constant16/1 -> Saturation Dynamic2/1
  Data Type Conversion18/1 -> ePWM6/1
  Data Type Conversion19/1 -> ePWM7/1
  Saturation Dynamic3/1 -> Data Type Conversion19/1
  Constant17/1 -> Saturation Dynamic2/3
  Saturation Dynamic2/1 -> Data Type Conversion18/1
  PWM1/1 -> Saturation Dynamic1/2
  PWM3/1 -> Saturation Dynamic3/2
  PWM2/1 -> Saturation Dynamic2/2
  From/1 -> ePWM5/2
  From1/1 -> ePWM6/2
  From2/1 -> ePWM7/2
  Trip/1 -> Gain/1
  Gain/1 -> Goto/1

== system AB_Final_of_MPC_Bandwidth_Result_UnbalancedNew/Subsystem1/Subsystem1 ==
  In1 : Inport
  In2 : Inport  Port=2
  Enable : EnablePort  StatesWhenEnabling=reset
  Add : Sum
  Add3 : Sum
  Bus Creator : BusCreator  Inputs=2
  Bus Selector1 : BusSelector  OutputSignals=signal1,signal2
  CodeGeneration : Subsystem  TreatAsAtomicUnit=on
  Constant3 : Constant  Value=100  OutDataTypeStr=single
  Counter Limited : simulink/Sources/Counter Limited  uplimit=599  tsamp=-1
  Data : Subsystem  TreatAsAtomicUnit=on
  Data_Conditioning : Subsystem
  End : Subsystem  TreatAsAtomicUnit=on
  Gain6 : Gain  Gain=1000  OutDataTypeStr=single
  Gain7 : Gain  Gain=1000  OutDataTypeStr=single
  If : If  IfExpression=u1 == 0  ElseIfExpressions=u1 == 599
  Merge : Merge  Inputs=3
  Merge1 : Merge  Inputs=3
  Mux : Mux  Inputs=2
  Mux1 : Mux  Inputs=2
  Start : Subsystem  TreatAsAtomicUnit=on
  Width : Width  OutDataTypeMode=All ports same datatype  DataType=uint16
  wires:
  Start/2(Iteration) -> Merge1/1
  Constant3/1 -> Add/2, Add3/1
  Counter Limited/1 -> If/1
  Data_Conditioning/1(Out1) -> Width/1, Start/1(Data), End/1(Data), Data/1(Data)
  End/1(Data_out) -> Merge/2
  End/2(Iteration) -> Merge1/2
  If/3 -> Data/Action
  Add/1 -> Gain6/1
  Data/2(Iteration) -> Merge1/3
  Merge1/1 -> Mux/2  "SCI_Tx_Iteration"
  Bus Selector1/1 -> Add/1  "<signal1>"
  Start/1(Data_out) -> Merge/1
  Add3/1 -> Gain7/1
  Mux1/1 -> Data_Conditioning/1(In1)
  In1/1 -> Bus Creator/1
  Merge/1 -> Mux/1  "SCI_Tx_Data"
  If/2 -> End/Action
  Data/1(Data_out) -> Merge/3
  Bus Creator/1 -> Bus Selector1/1
  Width/1 -> Start/2(Data_width), Data/2(Data_width), End/2(Data_width)
  Mux/1 -> CodeGeneration/1(Input)
  In2/1 -> Bus Creator/2
  Gain7/1 -> Mux1/2
  Bus Selector1/2 -> Add3/2  "<signal2>"
  If/1 -> Start/Action
  Gain6/1 -> Mux1/1

== system AB_Final_of_MPC_Bandwidth_Result_UnbalancedNew/Subsystem1/Subsystem2 ==
  In1 : Inport
  In2 : Inport  Port=2
  Enable : EnablePort  StatesWhenEnabling=reset
  Add : Sum
  Add3 : Sum
  Bus Creator : BusCreator  Inputs=2
  Bus Selector1 : BusSelector  OutputSignals=signal1,signal2
  CodeGeneration : Subsystem  TreatAsAtomicUnit=on
  Constant3 : Constant  Value=10  OutDataTypeStr=single
  Counter Limited : simulink/Sources/Counter Limited  uplimit=599  tsamp=-1
  Data : Subsystem  TreatAsAtomicUnit=on
  Data_Conditioning : Subsystem
  End : Subsystem  TreatAsAtomicUnit=on
  Gain6 : Gain  Gain=1000  OutDataTypeStr=single
  Gain7 : Gain  Gain=1000  OutDataTypeStr=single
  If : If  IfExpression=u1 == 0  ElseIfExpressions=u1 == 599
  Merge : Merge  Inputs=3
  Merge1 : Merge  Inputs=3
  Mux : Mux  Inputs=2
  Mux1 : Mux  Inputs=2
  Start : Subsystem  TreatAsAtomicUnit=on
  Width : Width  OutDataTypeMode=All ports same datatype  DataType=uint16
  wires:
  Start/2(Iteration) -> Merge1/1
  Constant3/1 -> Add/2, Add3/1
  Counter Limited/1 -> If/1
  Data_Conditioning/1(Out1) -> Width/1, Start/1(Data), End/1(Data), Data/1(Data)
  End/1(Data_out) -> Merge/2
  End/2(Iteration) -> Merge1/2
  If/3 -> Data/Action
  Add/1 -> Gain6/1
  Data/2(Iteration) -> Merge1/3
  Merge1/1 -> Mux/2  "SCI_Tx_Iteration"
  Bus Selector1/1 -> Add/1  "<signal1>"
  Start/1(Data_out) -> Merge/1
  Add3/1 -> Gain7/1
  Mux1/1 -> Data_Conditioning/1(In1)
  In1/1 -> Bus Creator/1
  Merge/1 -> Mux/1  "SCI_Tx_Data"
  If/2 -> End/Action
  Data/1(Data_out) -> Merge/3
  Bus Creator/1 -> Bus Selector1/1
  Width/1 -> Start/2(Data_width), Data/2(Data_width), End/2(Data_width)
  Mux/1 -> CodeGeneration/1(Input)
  In2/1 -> Bus Creator/2
  Gain7/1 -> Mux1/2
  Bus Selector1/2 -> Add3/2  "<signal2>"
  If/1 -> Start/Action
  Gain6/1 -> Mux1/1

== system AB_Final_of_MPC_Bandwidth_Result_UnbalancedNew/Subsystem1/Subsystem3 ==
  In1 : Inport
  Constant14 : Constant  Value=single(600)
  Gain26 : Gain  Gain=0
  IsNaN2 : RelationalOperator  Operator=isNaN  OutDataTypeStr=boolean  RndMeth=Simplest  InputSameDT=off
  Switch2 : Switch  SaturateOnIntegerOverflow=off  InputSameDT=off
  alpha : Outport
  wires:
  Switch2/1 -> alpha/1
  Constant14/1 -> Gain26/1
  IsNaN2/1 -> Switch2/2
  In1/1 -> Switch2/3, IsNaN2/1
  Gain26/1 -> Switch2/1

== system AB_Final_of_MPC_Bandwidth_Result_UnbalancedNew/Subsystem1/Subsystem4 ==
  In1 : Inport
  Constant14 : Constant  Value=single(600)
  Gain26 : Gain  Gain=0
  IsNaN2 : RelationalOperator  Operator=isNaN  OutDataTypeStr=boolean  RndMeth=Simplest  InputSameDT=off
  Switch2 : Switch  SaturateOnIntegerOverflow=off  InputSameDT=off
  beta : Outport
  wires:
  Switch2/1 -> beta/1
  Constant14/1 -> Gain26/1
  IsNaN2/1 -> Switch2/2
  In1/1 -> Switch2/3, IsNaN2/1
  Gain26/1 -> Switch2/1

== system AB_Final_of_MPC_Bandwidth_Result_UnbalancedNew/Subsystem1/Subsystem6 ==
  In1 : Inport
  In2 : Inport  Port=2
  theta : Inport  Port=3
  Add : Sum
  Add1 : Sum  Inputs=-+
  Cos : Trigonometry  Operator=cos
  Cos1 : Trigonometry
  From : From
  From4 : From
  Goto : Goto
  Product{,1..3} (4 alike) : Product
  Id : Outport
  Iq : Outport  Port=2
  wires:
  theta/1 -> Cos1/1, Cos/1
  In1/1 -> Goto/1
  In2/1 -> [b]
  From/1 -> Product/1
  Cos/1 -> [cosine]
  Cos1/1 -> [sinee]
  [cosine] -> Product/2
  [b] -> Product1/1
  [sinee] -> Product1/2
  Product/1 -> Add/1
  Product1/1 -> Add/2
  Add/1 -> Id/1
  [sinee] -> Product2/2
  [b] -> Product3/1
  Product3/1 -> Add1/2
  From4/1 -> Product2/1
  Product2/1 -> Add1/1
  [cosine] -> Product3/2
  Add1/1 -> Iq/1

== system AB_Final_of_MPC_Bandwidth_Result_UnbalancedNew/Subsystem1/System Outputs ==
